simulink model "Q2"  (R2022a)
settings: Solver=VariableStepAuto  StartTime=0.0  StopTime=40  RelTol=1e-3
libraries: simulink x2
settings Model: Creator=Hesam  LastModifiedBy=fatae
settings SolverCC: AlgebraicLoopSolver=TrustRegion
settings DebuggingCC: UnconnectedInputMsg=warning  UnconnectedOutputMsg=warning  UnconnectedLineMsg=warning  SFMachineParentedDataDiag=warning
settings SFSimCC: CustomCodeUndefinedFunction=UseInterfaceOnly

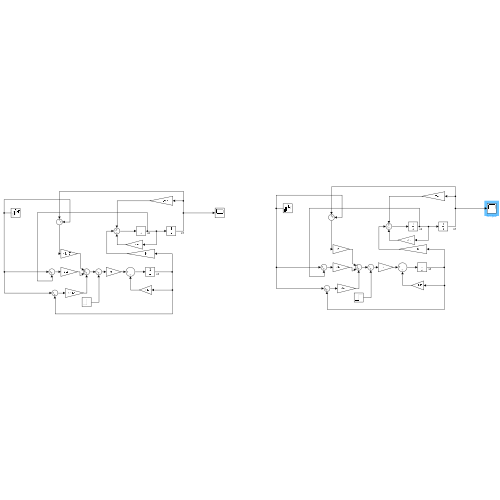
[thumbnail: Simulink's stored preview of the top-level diagram]
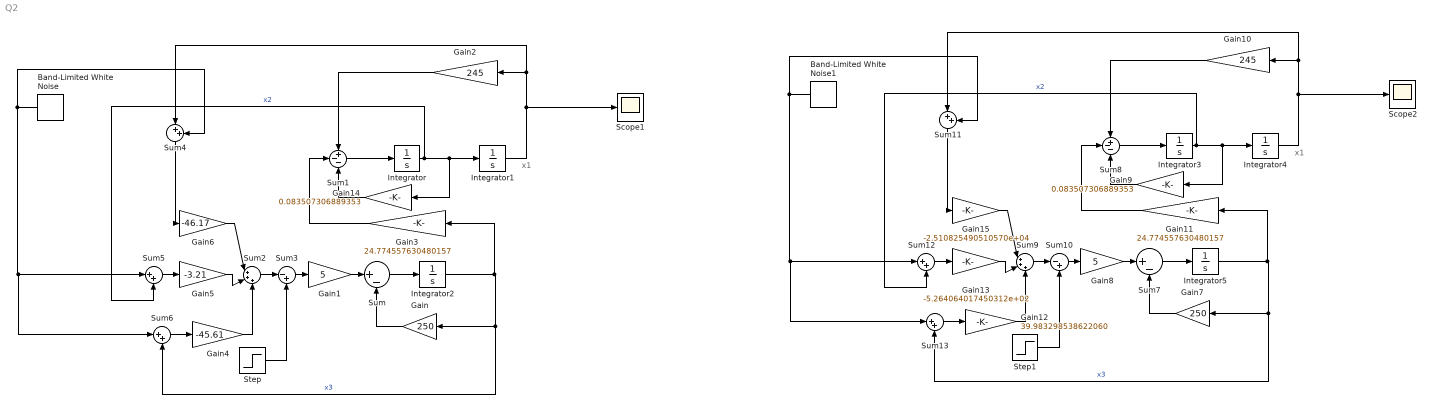
== system Q2 ==
  note: x1
  note: x1
  Band-Limited White Noise : simulink/Sources/Band-Limited White Noise  Cov=[0.01]  Ts=0.1  seed=[23341]
  Band-Limited White Noise1 : simulink/Sources/Band-Limited White Noise  Cov=[0.01]  Ts=0.1  seed=[23341]
  Gain : Gain  Gain=250
  Gain1 : Gain  Gain=5
  Gain10 : Gain  Gain=245
  Gain11 : Gain  Gain=24.774557630480157
  Gain12 : Gain  Gain=39.983298538622060
  Gain13 : Gain  Gain=-5.264064017450312e+02
  Gain14 : Gain  Gain=0.083507306889353
  Gain15 : Gain  Gain=-2.510825490510570e+04
  Gain2 : Gain  Gain=245
  Gain3 : Gain  Gain=24.774557630480157
  Gain4 : Gain  Gain=-45.61
  Gain5 : Gain  Gain=-3.21
  Gain6 : Gain  Gain=-46.17
  Gain7 : Gain  Gain=250
  Gain8 : Gain  Gain=5
  Gain9 : Gain  Gain=0.083507306889353
  Integrator{,1..5} (6 alike) : Integrator
  Scope1 : Scope
  Scope2 : Scope
  Step : Step  After=0.03  SampleTime=0
  Step1 : Step  After=0.03  SampleTime=0
  Sum : Sum  Inputs=|+-
  Sum1 : Sum  Inputs=+--
  Sum10 : Sum  Inputs=|-+
  Sum{4..6,11..13} (6 alike) : Sum  Inputs=|++
  Sum2 : Sum  Inputs=|+++
  Sum3 : Sum  Inputs=|-+
  Sum7 : Sum  Inputs=|+-
  Sum8 : Sum  Inputs=+--
  Sum9 : Sum  Inputs=|+++
  wires:
  Integrator/1 -> Integrator1/1, Gain14/1, Sum5/2  "x2"
  Sum/1 -> Integrator2/1
  Integrator2/1 -> Sum6/2, Gain/1, Gain3/1  "x3"
  Gain/1 -> Sum/2
  Gain1/1 -> Sum/1
  Sum1/1 -> Integrator/1
  Gain2/1 -> Sum1/1
  Gain3/1 -> Sum1/2
  Integrator1/1 -> Sum4/1, Gain2/1, Scope1/1
  Gain6/1 -> Sum2/1
  Gain5/1 -> Sum2/2
  Gain4/1 -> Sum2/3
  Sum2/1 -> Sum3/1
  Sum3/1 -> Gain1/1
  Step/1 -> Sum3/2
  Band-Limited White Noise/1 -> Sum4/2, Sum6/1, Sum5/1
  Sum4/1 -> Gain6/1
  Sum5/1 -> Gain5/1
  Sum6/1 -> Gain4/1
  Gain14/1 -> Sum1/3
  Gain9/1 -> Sum8/3
  Sum13/1 -> Gain12/1
  Sum11/1 -> Gain15/1
  Sum10/1 -> Gain8/1
  Sum8/1 -> Integrator3/1
  Gain13/1 -> Sum9/2
  Sum12/1 -> Gain13/1
  Step1/1 -> Sum10/2
  Gain12/1 -> Sum9/3
  Gain10/1 -> Sum8/1
  Integrator4/1 -> Sum11/1, Gain10/1, Scope2/1
  Band-Limited White Noise1/1 -> Sum11/2, Sum13/1, Sum12/1
  Sum9/1 -> Sum10/1
  Gain8/1 -> Sum7/1
  Gain7/1 -> Sum7/2
  Integrator5/1 -> Sum13/2, Gain7/1, Gain11/1  "x3"
  Gain15/1 -> Sum9/1
  Integrator3/1 -> Integrator4/1, Gain9/1, Sum12/2  "x2"
  Sum7/1 -> Integrator5/1
  Gain11/1 -> Sum8/2
